simulink model "if_test"  (Simulink 9.0)
settings: Solver=FixedStepAuto  StartTime=0.0  StopTime=1  FixedStep=1.000000  MaxStep=1  RelTol=1e-3  EnableMultiTasking=on
settings Model: SuppressorTable=22 serialization::archive 11 0 6 0 0 0 0 0  Creator=arnaud  LastModifiedBy=hbourbou
settings DataIOCC: LimitDataPoints=on  SaveFormat=Structure
settings DebuggingCC: UnderspecifiedInitializationDetection=Simplified  MergeDetectMultiDrivingBlocksExec=error  SolverPrmCheckMsg=warning
settings GRTTargetCC: GeneratePreprocessorConditionals=Disable all
settings ConfigComp: CovSFcnEnable=off

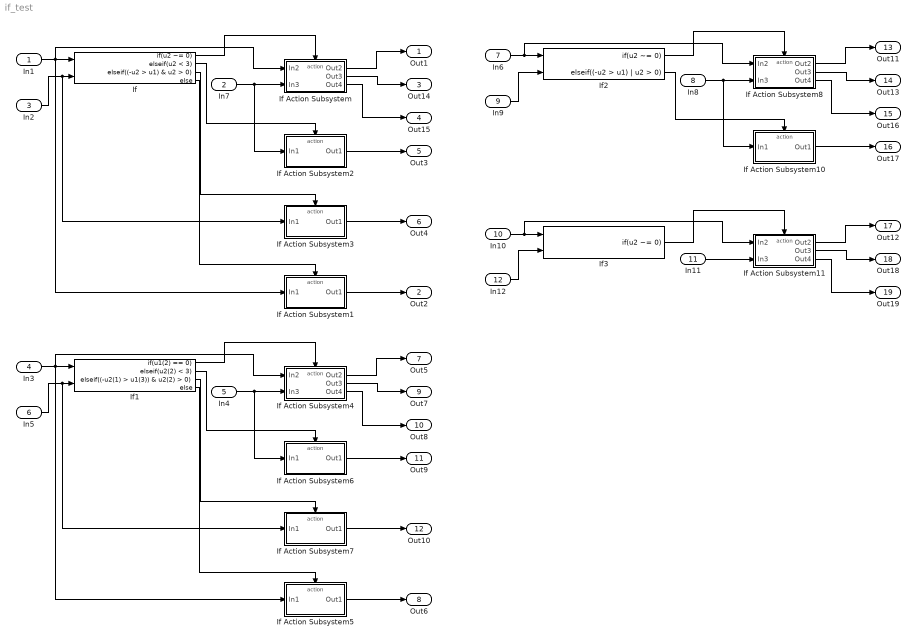
== system if_test ==
  In1 : Inport
  In7 : Inport  Port=2  OutDataTypeStr=boolean
  In2 : Inport  Port=3
  In3 : Inport  Port=4  PortDimensions=3
  In4 : Inport  Port=5  OutDataTypeStr=boolean
  In5 : Inport  Port=6  PortDimensions=4
  In6 : Inport  Port=7
  In8 : Inport  Port=8  OutDataTypeStr=boolean
  In9 : Inport  Port=9
  In10 : Inport  Port=10
  In11 : Inport  Port=11  OutDataTypeStr=boolean
  In12 : Inport  Port=12
  If : If  NumInputs=2  IfExpression=u2 ~= 0  ElseIfExpressions=u2 < 3, (-u2 > u1) & u2 > 0
  If Action Subsystem : Subsystem  TreatAsAtomicUnit=on
  If Action Subsystem1 : Subsystem  TreatAsAtomicUnit=on
  If Action Subsystem10 : Subsystem  TreatAsAtomicUnit=on
  If Action Subsystem11 : Subsystem  TreatAsAtomicUnit=on
  If Action Subsystem2 : Subsystem  TreatAsAtomicUnit=on
  If Action Subsystem3 : Subsystem  TreatAsAtomicUnit=on
  If Action Subsystem4 : Subsystem  TreatAsAtomicUnit=on
  If Action Subsystem5 : Subsystem  TreatAsAtomicUnit=on
  If Action Subsystem6 : Subsystem  TreatAsAtomicUnit=on
  If Action Subsystem7 : Subsystem  TreatAsAtomicUnit=on
  If Action Subsystem8 : Subsystem  TreatAsAtomicUnit=on
  If1 : If  NumInputs=2  IfExpression=u1(2) == 0  ElseIfExpressions=u2(2) < 3, (-u2(1) > u1(3)) & u2(2) > 0
  If2 : If  NumInputs=2  IfExpression=u2 ~= 0  ElseIfExpressions=(-u2 > u1) | u2 > 0  ShowElse=off
  If3 : If  NumInputs=2  IfExpression=u2 ~= 0  ShowElse=off
  Out1 : Outport
  Out2 : Outport  Port=2
  Out14 : Outport  Port=3
  Out15 : Outport  Port=4
  Out3 : Outport  Port=5
  Out4 : Outport  Port=6
  Out5 : Outport  Port=7
  Out6 : Outport  Port=8
  Out7 : Outport  Port=9
  Out8 : Outport  Port=10
  Out9 : Outport  Port=11
  Out10 : Outport  Port=12
  Out11 : Outport  Port=13
  Out13 : Outport  Port=14
  Out16 : Outport  Port=15
  Out17 : Outport  Port=16
  Out12 : Outport  Port=17
  Out18 : Outport  Port=18
  Out19 : Outport  Port=19
  wires:
  In1/1 -> If/1, If Action Subsystem1/1(In1), If Action Subsystem/1(In2)
  If/1 -> If Action Subsystem/Action
  If/4 -> If Action Subsystem1/Action
  If Action Subsystem/1(Out2) -> Out1/1
  If Action Subsystem1/1(Out1) -> Out2/1
  If Action Subsystem/2(Out3) -> Out14/1
  In7/1 -> If Action Subsystem2/1(In1), If Action Subsystem/2(In3)
  If Action Subsystem/3(Out4) -> Out15/1
  If Action Subsystem2/1(Out1) -> Out3/1
  If Action Subsystem3/1(Out1) -> Out4/1
  If/3 -> If Action Subsystem3/Action
  If/2 -> If Action Subsystem2/Action
  In2/1 -> If Action Subsystem3/1(In1), If/2
  In3/1 -> If1/1, If Action Subsystem5/1(In1), If Action Subsystem4/1(In2)
  If1/1 -> If Action Subsystem4/Action
  If1/4 -> If Action Subsystem5/Action
  If Action Subsystem4/1(Out2) -> Out5/1
  If Action Subsystem5/1(Out1) -> Out6/1
  If Action Subsystem4/2(Out3) -> Out7/1
  In4/1 -> If Action Subsystem6/1(In1), If Action Subsystem4/2(In3)
  If Action Subsystem4/3(Out4) -> Out8/1
  If Action Subsystem6/1(Out1) -> Out9/1
  If Action Subsystem7/1(Out1) -> Out10/1
  If1/3 -> If Action Subsystem7/Action
  If1/2 -> If Action Subsystem6/Action
  In5/1 -> If Action Subsystem7/1(In1), If1/2
  In6/1 -> If2/1, If Action Subsystem8/1(In2)
  If2/1 -> If Action Subsystem8/Action
  If Action Subsystem8/1(Out2) -> Out11/1
  If Action Subsystem8/2(Out3) -> Out13/1
  In8/1 -> If Action Subsystem10/1(In1), If Action Subsystem8/2(In3)
  If Action Subsystem8/3(Out4) -> Out16/1
  If Action Subsystem10/1(Out1) -> Out17/1
  If2/2 -> If Action Subsystem10/Action
  In9/1 -> If2/2
  In10/1 -> If3/1, If Action Subsystem11/1(In2)
  If3/1 -> If Action Subsystem11/Action
  If Action Subsystem11/1(Out2) -> Out12/1
  If Action Subsystem11/2(Out3) -> Out18/1
  In11/1 -> If Action Subsystem11/2(In3)
  If Action Subsystem11/3(Out4) -> Out19/1
  In12/1 -> If3/2

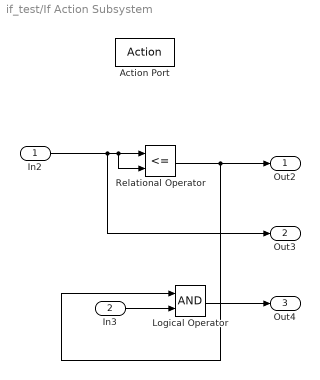
== system if_test/If Action Subsystem ==
  In2 : Inport
  In3 : Inport  Port=2
  Action Port : ActionPort  ActionType=then
  Logical Operator : Logic  AllPortsSameDT=off  OutDataTypeStr=boolean
  Relational Operator : RelationalOperator  Operator=<=  OutDataTypeStr=boolean  RndMeth=Nearest
  Out2 : Outport
  Out3 : Outport  Port=2
  Out4 : Outport  Port=3
  wires:
  In2/1 -> Relational Operator/1, Relational Operator/2, Out3/1
  Relational Operator/1 -> Logical Operator/1, Out2/1
  In3/1 -> Logical Operator/2
  Logical Operator/1 -> Out4/1

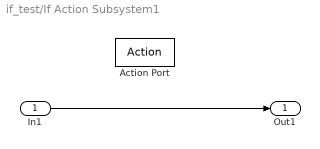
== system if_test/If Action Subsystem1 ==
  In1 : Inport
  Action Port : ActionPort  ActionType=else
  Out1 : Outport
  wires:
  In1/1 -> Out1/1

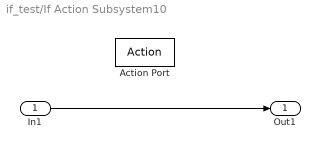
== system if_test/If Action Subsystem10 ==
  In1 : Inport
  Action Port : ActionPort  ActionType=elseif
  Out1 : Outport
  wires:
  In1/1 -> Out1/1

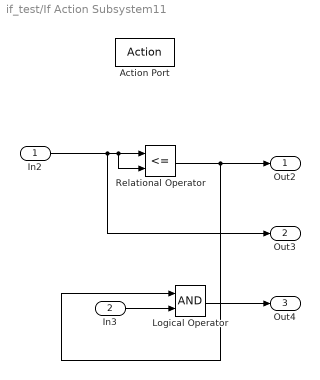
== system if_test/If Action Subsystem11 ==
  In2 : Inport
  In3 : Inport  Port=2
  Action Port : ActionPort  ActionType=then
  Logical Operator : Logic  AllPortsSameDT=off  OutDataTypeStr=boolean
  Relational Operator : RelationalOperator  Operator=<=  OutDataTypeStr=boolean  RndMeth=Nearest
  Out2 : Outport
  Out3 : Outport  Port=2
  Out4 : Outport  Port=3
  wires:
  In2/1 -> Relational Operator/1, Relational Operator/2, Out3/1
  Relational Operator/1 -> Logical Operator/1, Out2/1
  In3/1 -> Logical Operator/2
  Logical Operator/1 -> Out4/1

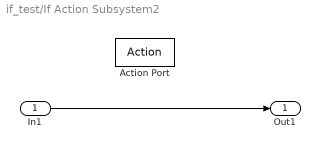
== system if_test/If Action Subsystem2 ==
  In1 : Inport
  Action Port : ActionPort  ActionType=elseif
  Out1 : Outport
  wires:
  In1/1 -> Out1/1

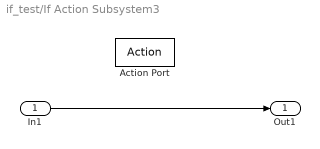
== system if_test/If Action Subsystem3 ==
  In1 : Inport
  Action Port : ActionPort  ActionType=elseif
  Out1 : Outport
  wires:
  In1/1 -> Out1/1

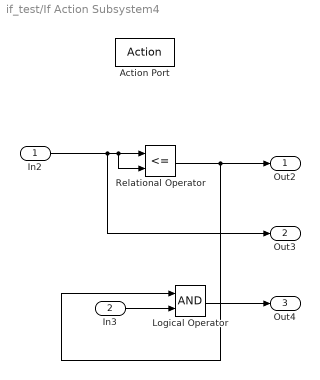
== system if_test/If Action Subsystem4 ==
  In2 : Inport
  In3 : Inport  Port=2
  Action Port : ActionPort  ActionType=then
  Logical Operator : Logic  AllPortsSameDT=off  OutDataTypeStr=boolean
  Relational Operator : RelationalOperator  Operator=<=  OutDataTypeStr=boolean  RndMeth=Nearest
  Out2 : Outport
  Out3 : Outport  Port=2
  Out4 : Outport  Port=3
  wires:
  In2/1 -> Relational Operator/1, Relational Operator/2, Out3/1
  Relational Operator/1 -> Logical Operator/1, Out2/1
  In3/1 -> Logical Operator/2
  Logical Operator/1 -> Out4/1

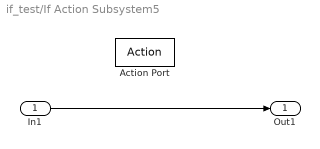
== system if_test/If Action Subsystem5 ==
  In1 : Inport
  Action Port : ActionPort  ActionType=else
  Out1 : Outport
  wires:
  In1/1 -> Out1/1

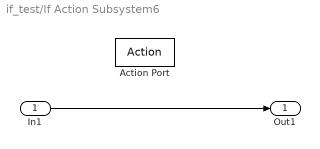
== system if_test/If Action Subsystem6 ==
  In1 : Inport
  Action Port : ActionPort  ActionType=elseif
  Out1 : Outport
  wires:
  In1/1 -> Out1/1

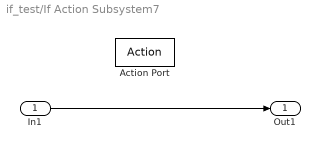
== system if_test/If Action Subsystem7 ==
  In1 : Inport
  Action Port : ActionPort  ActionType=elseif
  Out1 : Outport
  wires:
  In1/1 -> Out1/1

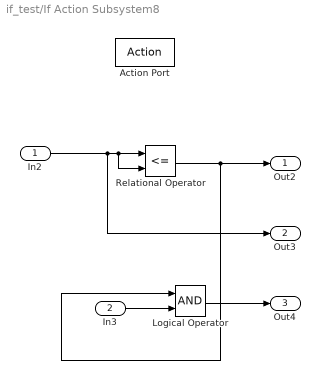
== system if_test/If Action Subsystem8 ==
  In2 : Inport
  In3 : Inport  Port=2
  Action Port : ActionPort  ActionType=then
  Logical Operator : Logic  AllPortsSameDT=off  OutDataTypeStr=boolean
  Relational Operator : RelationalOperator  Operator=<=  OutDataTypeStr=boolean  RndMeth=Nearest
  Out2 : Outport
  Out3 : Outport  Port=2
  Out4 : Outport  Port=3
  wires:
  In2/1 -> Relational Operator/1, Relational Operator/2, Out3/1
  Relational Operator/1 -> Logical Operator/1, Out2/1
  In3/1 -> Logical Operator/2
  Logical Operator/1 -> Out4/1
